simulink model "c00004M_harness"  (R2018a)
settings: Solver=ode3  StartTime=0.0  StopTime=10.0  RelTol=1e-3  EnableMultiTasking=on
undefined symbols (not defined in the file): b, DiscIntNeverNeededParam, J, K, L, PosMinimaW3, PosMinimaW4, R, sigbuilder_block
(part 22 of 74)

== system c00004M_harness/M132/Cyber ==
  note: Sensors
  note: Inputs For Window1
  note: Inputs for Window 2
  note: Inputs for window 3
  note: Inputs for window 4
  note: Users
  note: Users
  note: Sensors
  note: Users
  note: Sensors
  note: Users
  note: Sensors
  note: USERS
      | ---------------------------------
      | 0: None
      | 1: Ventana Arriba
      | 2: Ventana hasta arriba
      | 3: Ventana abajo
      | 4: Ventana hasta abajo
  note: 1: SUBE
      | 0: PARADO
      | -1 BAJA
  note: D = Driver (W1)
      | P1 = Passenger 1 (W2)
      | P2 = Passenger 2 (W3)
      | P3 = Passenger 3 (W4)
      | O = Obstacle
      | C = Control
      | Pri = Prioritizer
      | LD = LockDriver
      | PosW = PositionWindow
      | WL = WindowLogic
      | OW = ObstacleWindow
      | CWXC = ControlWindowXCentralized
      | S = Sensor
      | L = Lock
      | WPos = WindowPosition
      | M = Memory
      | InW = InputWindow
      | WIn = WindowInput
  PosW1 : Inport
  PosW2 : Inport  Port=2
  PosW3 : Inport  Port=3
  PosW4 : Inport  Port=4
  DW1 : Inport  Port=5
  DW3 : Inport  Port=6
  DW4 : Inport  Port=7
  P1W2 : Inport  Port=8
  P2W3 : Inport  Port=9
  P1W3 : Inport  Port=10
  P3W4 : Inport  Port=11
  P1W4 : Inport  Port=12
  OW1 : Inport  Port=13
  OW2 : Inport  Port=14
  OW3 : Inport  Port=15
  OW4 : Inport  Port=16
  CW1C : Inport  Port=17
  CW3C : Inport  Port=18
  CW4C : Inport  Port=19
  Pri1 : Subsystem
  Pri3 : Subsystem
  Pri4 : Subsystem
  WL : Subsystem
  WL1 : Subsystem
  WL2 : Subsystem
  WL3 : Subsystem
  W1 : Outport
  W2 : Outport  Port=2
  W3 : Outport  Port=3
  W4 : Outport  Port=4
  wires:
  CW4C/1 -> Pri4/4(CW4C)
  CW3C/1 -> Pri1/4(CW3C)
  CW1C/1 -> Pri3/2(CW1C)
  Pri3/1(User) -> WL/2(User)
  WL3/1(WindowLogicOutput) -> W4/1
  WL2/1(WindowLogicOutput) -> W3/1
  Pri4/1(User) -> WL3/2(User)
  OW4/1 -> WL3/3(OW)
  PosW4/1 -> WL3/1(WPos)
  P1W4/1 -> Pri4/3(P1)
  P3W4/1 -> Pri4/2(P)
  DW4/1 -> Pri4/1(D)
  P1W3/1 -> Pri1/3(P1)
  P2W3/1 -> Pri1/2(P)
  DW3/1 -> Pri1/1(D)
  OW3/1 -> WL2/3(OW)
  PosW3/1 -> WL2/1(WPos)
  Pri1/1(User) -> WL2/2(User)
  WL1/1(WindowLogicOutput) -> W2/1
  OW2/1 -> WL1/3(OW)
  PosW2/1 -> WL1/1(WPos)
  WL/1(WindowLogicOutput) -> W1/1
  DW1/1 -> Pri3/1(D)
  OW1/1 -> WL/3(OW)
  PosW1/1 -> WL/1(WPos)
  P1W2/1 -> WL1/2(User)

== system c00004M_harness/M132/Physical ==
  InW1 : Inport
  InW2 : Inport  Port=2
  InW3 : Inport  Port=3
  InW4 : Inport  Port=4
  W : Subsystem
  W5 : Subsystem
  W6 : Subsystem
  W7 : Subsystem
  W1 : Outport
  W2 : Outport  Port=2
  W3 : Outport  Port=3
  W4 : Outport  Port=4
  wires:
  W7/1(WPos) -> W4/1
  W6/1(WPos) -> W3/1
  W5/1(WPos) -> W2/1
  W/1(WPos) -> W1/1
  InW4/1 -> W7/1(WIn)
  InW3/1 -> W6/1(WIn)
  InW2/1 -> W5/1(WIn)
  InW1/1 -> W/1(WIn)

== system c00004M_harness/M132/S1 ==
  PhyMeasure : Inport
  SensorOut : Outport
  wires:
  PhyMeasure/1 -> SensorOut/1

== system c00004M_harness/M132/S2 ==
  PhyMeasure : Inport
  SensorOut : Outport
  wires:
  PhyMeasure/1 -> SensorOut/1

== system c00004M_harness/M132/S3 ==
  PhyMeasure : Inport
  SensorOut : Outport
  wires:
  PhyMeasure/1 -> SensorOut/1

== system c00004M_harness/M132/S4 ==
  PhyMeasure : Inport
  SensorOut : Outport
  wires:
  PhyMeasure/1 -> SensorOut/1

== system c00004M_harness/M133/Cyber ==
  note: Sensors
  note: Inputs For Window1
  note: Inputs for Window 2
  note: Inputs for window 3
  note: Inputs for window 4
  note: Users
  note: Users
  note: Sensors
  note: Users
  note: Sensors
  note: Users
  note: Sensors
  note: USERS
      | ---------------------------------
      | 0: None
      | 1: Ventana Arriba
      | 2: Ventana hasta arriba
      | 3: Ventana abajo
      | 4: Ventana hasta abajo
  note: 1: SUBE
      | 0: PARADO
      | -1 BAJA
  note: D = Driver (W1)
      | P1 = Passenger 1 (W2)
      | P2 = Passenger 2 (W3)
      | P3 = Passenger 3 (W4)
      | O = Obstacle
      | C = Control
      | Pri = Prioritizer
      | LD = LockDriver
      | PosW = PositionWindow
      | WL = WindowLogic
      | OW = ObstacleWindow
      | CWXC = ControlWindowXCentralized
      | S = Sensor
      | L = Lock
      | WPos = WindowPosition
      | M = Memory
      | InW = InputWindow
      | WIn = WindowInput
  PosW1 : Inport
  PosW2 : Inport  Port=2
  PosW3 : Inport  Port=3
  PosW4 : Inport  Port=4
  DW1 : Inport  Port=5
  DW3 : Inport  Port=6
  DW4 : Inport  Port=7
  P1W2 : Inport  Port=8
  P2W3 : Inport  Port=9
  P1W3 : Inport  Port=10
  P3W4 : Inport  Port=11
  P1W4 : Inport  Port=12
  OW1 : Inport  Port=13
  OW2 : Inport  Port=14
  OW3 : Inport  Port=15
  OW4 : Inport  Port=16
  CW1C : Inport  Port=17
  CW3C : Inport  Port=18
  CW4C : Inport  Port=19
  Pri1 : Subsystem
  Pri3 : Subsystem
  Pri4 : Subsystem
  WL : Subsystem
  WL1 : Subsystem
  WL2 : Subsystem
  WL3 : Subsystem
  W1 : Outport
  W2 : Outport  Port=2
  W3 : Outport  Port=3
  W4 : Outport  Port=4
  wires:
  CW4C/1 -> Pri4/4(CW4C)
  CW3C/1 -> Pri1/4(CW3C)
  CW1C/1 -> Pri3/2(CW1C)
  Pri3/1(User) -> WL/2(User)
  WL3/1(WindowLogicOutput) -> W4/1
  WL2/1(WindowLogicOutput) -> W3/1
  Pri4/1(User) -> WL3/2(User)
  OW4/1 -> WL3/3(OW)
  PosW4/1 -> WL3/1(WPos)
  P1W4/1 -> Pri4/3(P1)
  P3W4/1 -> Pri4/2(P)
  DW4/1 -> Pri4/1(D)
  P1W3/1 -> Pri1/3(P1)
  P2W3/1 -> Pri1/2(P)
  DW3/1 -> Pri1/1(D)
  OW3/1 -> WL2/3(OW)
  PosW3/1 -> WL2/1(WPos)
  Pri1/1(User) -> WL2/2(User)
  WL1/1(WindowLogicOutput) -> W2/1
  OW2/1 -> WL1/3(OW)
  PosW2/1 -> WL1/1(WPos)
  WL/1(WindowLogicOutput) -> W1/1
  DW1/1 -> Pri3/1(D)
  OW1/1 -> WL/3(OW)
  PosW1/1 -> WL/1(WPos)
  P1W2/1 -> WL1/2(User)

== system c00004M_harness/M133/Physical ==
  InW1 : Inport
  InW2 : Inport  Port=2
  InW3 : Inport  Port=3
  InW4 : Inport  Port=4
  W : Subsystem
  W5 : Subsystem
  W6 : Subsystem
  W7 : Subsystem
  W1 : Outport
  W2 : Outport  Port=2
  W3 : Outport  Port=3
  W4 : Outport  Port=4
  wires:
  W7/1(WPos) -> W4/1
  W6/1(WPos) -> W3/1
  W5/1(WPos) -> W2/1
  W/1(WPos) -> W1/1
  InW4/1 -> W7/1(WIn)
  InW3/1 -> W6/1(WIn)
  InW2/1 -> W5/1(WIn)
  InW1/1 -> W/1(WIn)

== system c00004M_harness/M133/S1 ==
  PhyMeasure : Inport
  SensorOut : Outport
  wires:
  PhyMeasure/1 -> SensorOut/1

== system c00004M_harness/M133/S2 ==
  PhyMeasure : Inport
  SensorOut : Outport
  wires:
  PhyMeasure/1 -> SensorOut/1

== system c00004M_harness/M133/S3 ==
  PhyMeasure : Inport
  SensorOut : Outport
  wires:
  PhyMeasure/1 -> SensorOut/1

== system c00004M_harness/M133/S4 ==
  PhyMeasure : Inport
  SensorOut : Outport
  wires:
  PhyMeasure/1 -> SensorOut/1

== system c00004M_harness/M134/Cyber ==
  note: Sensors
  note: Inputs For Window1
  note: Inputs for Window 2
  note: Inputs for window 3
  note: Inputs for window 4
  note: Users
  note: Users
  note: Sensors
  note: Users
  note: Sensors
  note: Users
  note: Sensors
  note: USERS
      | ---------------------------------
      | 0: None
      | 1: Ventana Arriba
      | 2: Ventana hasta arriba
      | 3: Ventana abajo
      | 4: Ventana hasta abajo
  note: 1: SUBE
      | 0: PARADO
      | -1 BAJA
  note: D = Driver (W1)
      | P1 = Passenger 1 (W2)
      | P2 = Passenger 2 (W3)
      | P3 = Passenger 3 (W4)
      | O = Obstacle
      | C = Control
      | Pri = Prioritizer
      | LD = LockDriver
      | PosW = PositionWindow
      | WL = WindowLogic
      | OW = ObstacleWindow
      | CWXC = ControlWindowXCentralized
      | S = Sensor
      | L = Lock
      | WPos = WindowPosition
      | M = Memory
      | InW = InputWindow
      | WIn = WindowInput
  PosW1 : Inport
  PosW2 : Inport  Port=2
  PosW3 : Inport  Port=3
  PosW4 : Inport  Port=4
  DW1 : Inport  Port=5
  DW3 : Inport  Port=6
  DW4 : Inport  Port=7
  P1W2 : Inport  Port=8
  P2W3 : Inport  Port=9
  P1W3 : Inport  Port=10
  P3W4 : Inport  Port=11
  P1W4 : Inport  Port=12
  OW1 : Inport  Port=13
  OW2 : Inport  Port=14
  OW3 : Inport  Port=15
  OW4 : Inport  Port=16
  CW1C : Inport  Port=17
  CW3C : Inport  Port=18
  CW4C : Inport  Port=19
  Pri1 : Subsystem
  Pri3 : Subsystem
  Pri4 : Subsystem
  WL : Subsystem
  WL1 : Subsystem
  WL2 : Subsystem
  WL3 : Subsystem
  W1 : Outport
  W2 : Outport  Port=2
  W3 : Outport  Port=3
  W4 : Outport  Port=4
  wires:
  CW4C/1 -> Pri4/4(CW4C)
  CW3C/1 -> Pri1/4(CW3C)
  CW1C/1 -> Pri3/2(CW1C)
  Pri3/1(User) -> WL/2(User)
  WL3/1(WindowLogicOutput) -> W4/1
  WL2/1(WindowLogicOutput) -> W3/1
  Pri4/1(User) -> WL3/2(User)
  OW4/1 -> WL3/3(OW)
  PosW4/1 -> WL3/1(WPos)
  P1W4/1 -> Pri4/3(P1)
  P3W4/1 -> Pri4/2(P)
  DW4/1 -> Pri4/1(D)
  P1W3/1 -> Pri1/3(P1)
  P2W3/1 -> Pri1/2(P)
  DW3/1 -> Pri1/1(D)
  OW3/1 -> WL2/3(OW)
  PosW3/1 -> WL2/1(WPos)
  Pri1/1(User) -> WL2/2(User)
  WL1/1(WindowLogicOutput) -> W2/1
  OW2/1 -> WL1/3(OW)
  PosW2/1 -> WL1/1(WPos)
  WL/1(WindowLogicOutput) -> W1/1
  DW1/1 -> Pri3/1(D)
  OW1/1 -> WL/3(OW)
  PosW1/1 -> WL/1(WPos)
  P1W2/1 -> WL1/2(User)

== system c00004M_harness/M134/Physical ==
  InW1 : Inport
  InW2 : Inport  Port=2
  InW3 : Inport  Port=3
  InW4 : Inport  Port=4
  W : Subsystem
  W5 : Subsystem
  W6 : Subsystem
  W7 : Subsystem
  W1 : Outport
  W2 : Outport  Port=2
  W3 : Outport  Port=3
  W4 : Outport  Port=4
  wires:
  W7/1(WPos) -> W4/1
  W6/1(WPos) -> W3/1
  W5/1(WPos) -> W2/1
  W/1(WPos) -> W1/1
  InW4/1 -> W7/1(WIn)
  InW3/1 -> W6/1(WIn)
  InW2/1 -> W5/1(WIn)
  InW1/1 -> W/1(WIn)

== system c00004M_harness/M134/S1 ==
  PhyMeasure : Inport
  SensorOut : Outport
  wires:
  PhyMeasure/1 -> SensorOut/1

== system c00004M_harness/M134/S2 ==
  PhyMeasure : Inport
  SensorOut : Outport
  wires:
  PhyMeasure/1 -> SensorOut/1

== system c00004M_harness/M134/S3 ==
  PhyMeasure : Inport
  SensorOut : Outport
  wires:
  PhyMeasure/1 -> SensorOut/1

== system c00004M_harness/M134/S4 ==
  PhyMeasure : Inport
  SensorOut : Outport
  wires:
  PhyMeasure/1 -> SensorOut/1

== system c00004M_harness/M135/Cyber ==
  note: Sensors
  note: Inputs For Window1
  note: Inputs for Window 2
  note: Inputs for window 3
  note: Inputs for window 4
  note: Users
  note: Users
  note: Sensors
  note: Users
  note: Sensors
  note: Users
  note: Sensors
  note: USERS
      | ---------------------------------
      | 0: None
      | 1: Ventana Arriba
      | 2: Ventana hasta arriba
      | 3: Ventana abajo
      | 4: Ventana hasta abajo
  note: 1: SUBE
      | 0: PARADO
      | -1 BAJA
  note: D = Driver (W1)
      | P1 = Passenger 1 (W2)
      | P2 = Passenger 2 (W3)
      | P3 = Passenger 3 (W4)
      | O = Obstacle
      | C = Control
      | Pri = Prioritizer
      | LD = LockDriver
      | PosW = PositionWindow
      | WL = WindowLogic
      | OW = ObstacleWindow
      | CWXC = ControlWindowXCentralized
      | S = Sensor
      | L = Lock
      | WPos = WindowPosition
      | M = Memory
      | InW = InputWindow
      | WIn = WindowInput
  PosW1 : Inport
  PosW2 : Inport  Port=2
  PosW3 : Inport  Port=3
  PosW4 : Inport  Port=4
  DW1 : Inport  Port=5
  DW3 : Inport  Port=6
  DW4 : Inport  Port=7
  P1W2 : Inport  Port=8
  P2W3 : Inport  Port=9
  P1W3 : Inport  Port=10
  P3W4 : Inport  Port=11
  P1W4 : Inport  Port=12
  OW1 : Inport  Port=13
  OW2 : Inport  Port=14
  OW3 : Inport  Port=15
  OW4 : Inport  Port=16
  CW1C : Inport  Port=17
  CW3C : Inport  Port=18
  CW4C : Inport  Port=19
  Pri1 : Subsystem
  Pri3 : Subsystem
  Pri4 : Subsystem
  WL : Subsystem
  WL1 : Subsystem
  WL2 : Subsystem
  WL3 : Subsystem
  W1 : Outport
  W2 : Outport  Port=2
  W3 : Outport  Port=3
  W4 : Outport  Port=4
  wires:
  CW4C/1 -> Pri4/4(CW4C)
  CW3C/1 -> Pri1/4(CW3C)
  CW1C/1 -> Pri3/2(CW1C)
  Pri3/1(User) -> WL/2(User)
  WL3/1(WindowLogicOutput) -> W4/1
  WL2/1(WindowLogicOutput) -> W3/1
  Pri4/1(User) -> WL3/2(User)
  OW4/1 -> WL3/3(OW)
  PosW4/1 -> WL3/1(WPos)
  P1W4/1 -> Pri4/3(P1)
  P3W4/1 -> Pri4/2(P)
  DW4/1 -> Pri4/1(D)
  P1W3/1 -> Pri1/3(P1)
  P2W3/1 -> Pri1/2(P)
  DW3/1 -> Pri1/1(D)
  OW3/1 -> WL2/3(OW)
  PosW3/1 -> WL2/1(WPos)
  Pri1/1(User) -> WL2/2(User)
  WL1/1(WindowLogicOutput) -> W2/1
  OW2/1 -> WL1/3(OW)
  PosW2/1 -> WL1/1(WPos)
  WL/1(WindowLogicOutput) -> W1/1
  DW1/1 -> Pri3/1(D)
  OW1/1 -> WL/3(OW)
  PosW1/1 -> WL/1(WPos)
  P1W2/1 -> WL1/2(User)

== system c00004M_harness/M135/Physical ==
  InW1 : Inport
  InW2 : Inport  Port=2
  InW3 : Inport  Port=3
  InW4 : Inport  Port=4
  W : Subsystem
  W5 : Subsystem
  W6 : Subsystem
  W7 : Subsystem
  W1 : Outport
  W2 : Outport  Port=2
  W3 : Outport  Port=3
  W4 : Outport  Port=4
  wires:
  W7/1(WPos) -> W4/1
  W6/1(WPos) -> W3/1
  W5/1(WPos) -> W2/1
  W/1(WPos) -> W1/1
  InW4/1 -> W7/1(WIn)
  InW3/1 -> W6/1(WIn)
  InW2/1 -> W5/1(WIn)
  InW1/1 -> W/1(WIn)

== system c00004M_harness/M135/S1 ==
  PhyMeasure : Inport
  SensorOut : Outport
  wires:
  PhyMeasure/1 -> SensorOut/1

== system c00004M_harness/M135/S2 ==
  PhyMeasure : Inport
  SensorOut : Outport
  wires:
  PhyMeasure/1 -> SensorOut/1

== system c00004M_harness/M135/S3 ==
  PhyMeasure : Inport
  SensorOut : Outport
  wires:
  PhyMeasure/1 -> SensorOut/1

== system c00004M_harness/M135/S4 ==
  PhyMeasure : Inport
  SensorOut : Outport
  wires:
  PhyMeasure/1 -> SensorOut/1

== system c00004M_harness/M136/Cyber ==
  note: Sensors
  note: Inputs For Window1
  note: Inputs for Window 2
  note: Inputs for window 3
  note: Inputs for window 4
  note: Users
  note: Users
  note: Sensors
  note: Users
  note: Sensors
  note: Users
  note: Sensors
  note: USERS
      | ---------------------------------
      | 0: None
      | 1: Ventana Arriba
      | 2: Ventana hasta arriba
      | 3: Ventana abajo
      | 4: Ventana hasta abajo
  note: 1: SUBE
      | 0: PARADO
      | -1 BAJA
  note: D = Driver (W1)
      | P1 = Passenger 1 (W2)
      | P2 = Passenger 2 (W3)
      | P3 = Passenger 3 (W4)
      | O = Obstacle
      | C = Control
      | Pri = Prioritizer
      | LD = LockDriver
      | PosW = PositionWindow
      | WL = WindowLogic
      | OW = ObstacleWindow
      | CWXC = ControlWindowXCentralized
      | S = Sensor
      | L = Lock
      | WPos = WindowPosition
      | M = Memory
      | InW = InputWindow
      | WIn = WindowInput
  PosW1 : Inport
  PosW2 : Inport  Port=2
  PosW3 : Inport  Port=3
  PosW4 : Inport  Port=4
  DW1 : Inport  Port=5
  DW3 : Inport  Port=6
  DW4 : Inport  Port=7
  P1W2 : Inport  Port=8
  P2W3 : Inport  Port=9
  P1W3 : Inport  Port=10
  P3W4 : Inport  Port=11
  P1W4 : Inport  Port=12
  OW1 : Inport  Port=13
  OW2 : Inport  Port=14
  OW3 : Inport  Port=15
  OW4 : Inport  Port=16
  CW1C : Inport  Port=17
  CW3C : Inport  Port=18
  CW4C : Inport  Port=19
  Pri1 : Subsystem
  Pri3 : Subsystem
  Pri4 : Subsystem
  WL : Subsystem
  WL1 : Subsystem
  WL2 : Subsystem
  WL3 : Subsystem
  W1 : Outport
  W2 : Outport  Port=2
  W3 : Outport  Port=3
  W4 : Outport  Port=4
  wires:
  CW4C/1 -> Pri4/4(CW4C)
  CW3C/1 -> Pri1/4(CW3C)
  CW1C/1 -> Pri3/2(CW1C)
  Pri3/1(User) -> WL/2(User)
  WL3/1(WindowLogicOutput) -> W4/1
  WL2/1(WindowLogicOutput) -> W3/1
  Pri4/1(User) -> WL3/2(User)
  OW4/1 -> WL3/3(OW)
  PosW4/1 -> WL3/1(WPos)
  P1W4/1 -> Pri4/3(P1)
  P3W4/1 -> Pri4/2(P)
  DW4/1 -> Pri4/1(D)
  P1W3/1 -> Pri1/3(P1)
  P2W3/1 -> Pri1/2(P)
  DW3/1 -> Pri1/1(D)
  OW3/1 -> WL2/3(OW)
  PosW3/1 -> WL2/1(WPos)
  Pri1/1(User) -> WL2/2(User)
  WL1/1(WindowLogicOutput) -> W2/1
  OW2/1 -> WL1/3(OW)
  PosW2/1 -> WL1/1(WPos)
  WL/1(WindowLogicOutput) -> W1/1
  DW1/1 -> Pri3/1(D)
  OW1/1 -> WL/3(OW)
  PosW1/1 -> WL/1(WPos)
  P1W2/1 -> WL1/2(User)

== system c00004M_harness/M136/Physical ==
  InW1 : Inport
  InW2 : Inport  Port=2
  InW3 : Inport  Port=3
  InW4 : Inport  Port=4
  W : Subsystem
  W5 : Subsystem
  W6 : Subsystem
  W7 : Subsystem
  W1 : Outport
  W2 : Outport  Port=2
  W3 : Outport  Port=3
  W4 : Outport  Port=4
  wires:
  W7/1(WPos) -> W4/1
  W6/1(WPos) -> W3/1
  W5/1(WPos) -> W2/1
  W/1(WPos) -> W1/1
  InW4/1 -> W7/1(WIn)
  InW3/1 -> W6/1(WIn)
  InW2/1 -> W5/1(WIn)
  InW1/1 -> W/1(WIn)

== system c00004M_harness/M136/S1 ==
  PhyMeasure : Inport
  SensorOut : Outport
  wires:
  PhyMeasure/1 -> SensorOut/1

== system c00004M_harness/M136/S2 ==
  PhyMeasure : Inport
  SensorOut : Outport
  wires:
  PhyMeasure/1 -> SensorOut/1

== system c00004M_harness/M136/S3 ==
  PhyMeasure : Inport
  SensorOut : Outport
  wires:
  PhyMeasure/1 -> SensorOut/1

== system c00004M_harness/M136/S4 ==
  PhyMeasure : Inport
  SensorOut : Outport
  wires:
  PhyMeasure/1 -> SensorOut/1

== system c00004M_harness/M137/Cyber ==
  note: Sensors
  note: Inputs For Window1
  note: Inputs for Window 2
  note: Inputs for window 3
  note: Inputs for window 4
  note: Users
  note: Users
  note: Sensors
  note: Users
  note: Sensors
  note: Users
  note: Sensors
  note: USERS
      | ---------------------------------
      | 0: None
      | 1: Ventana Arriba
      | 2: Ventana hasta arriba
      | 3: Ventana abajo
      | 4: Ventana hasta abajo
  note: 1: SUBE
      | 0: PARADO
      | -1 BAJA
  note: D = Driver (W1)
      | P1 = Passenger 1 (W2)
      | P2 = Passenger 2 (W3)
      | P3 = Passenger 3 (W4)
      | O = Obstacle
      | C = Control
      | Pri = Prioritizer
      | LD = LockDriver
      | PosW = PositionWindow
      | WL = WindowLogic
      | OW = ObstacleWindow
      | CWXC = ControlWindowXCentralized
      | S = Sensor
      | L = Lock
      | WPos = WindowPosition
      | M = Memory
      | InW = InputWindow
      | WIn = WindowInput
  PosW1 : Inport
  PosW2 : Inport  Port=2
  PosW3 : Inport  Port=3
  PosW4 : Inport  Port=4
  DW1 : Inport  Port=5
  DW3 : Inport  Port=6
  DW4 : Inport  Port=7
  P1W2 : Inport  Port=8
  P2W3 : Inport  Port=9
  P1W3 : Inport  Port=10
  P3W4 : Inport  Port=11
  P1W4 : Inport  Port=12
  OW1 : Inport  Port=13
  OW2 : Inport  Port=14
  OW3 : Inport  Port=15
  OW4 : Inport  Port=16
  CW1C : Inport  Port=17
  CW3C : Inport  Port=18
  CW4C : Inport  Port=19
  Pri1 : Subsystem
  Pri3 : Subsystem
  Pri4 : Subsystem
  WL : Subsystem
  WL1 : Subsystem
  WL2 : Subsystem
  WL3 : Subsystem
  W1 : Outport
  W2 : Outport  Port=2
  W3 : Outport  Port=3
  W4 : Outport  Port=4
  wires:
  CW4C/1 -> Pri4/4(CW4C)
  CW3C/1 -> Pri1/4(CW3C)
  CW1C/1 -> Pri3/2(CW1C)
  Pri3/1(User) -> WL/2(User)
  WL3/1(WindowLogicOutput) -> W4/1
  WL2/1(WindowLogicOutput) -> W3/1
  Pri4/1(User) -> WL3/2(User)
  OW4/1 -> WL3/3(OW)
  PosW4/1 -> WL3/1(WPos)
  P1W4/1 -> Pri4/3(P1)
  P3W4/1 -> Pri4/2(P)
  DW4/1 -> Pri4/1(D)
  P1W3/1 -> Pri1/3(P1)
  P2W3/1 -> Pri1/2(P)
  DW3/1 -> Pri1/1(D)
  OW3/1 -> WL2/3(OW)
  PosW3/1 -> WL2/1(WPos)
  Pri1/1(User) -> WL2/2(User)
  WL1/1(WindowLogicOutput) -> W2/1
  OW2/1 -> WL1/3(OW)
  PosW2/1 -> WL1/1(WPos)
  WL/1(WindowLogicOutput) -> W1/1
  DW1/1 -> Pri3/1(D)
  OW1/1 -> WL/3(OW)
  PosW1/1 -> WL/1(WPos)
  P1W2/1 -> WL1/2(User)

== system c00004M_harness/M137/Physical ==
  InW1 : Inport
  InW2 : Inport  Port=2
  InW3 : Inport  Port=3
  InW4 : Inport  Port=4
  W : Subsystem
  W5 : Subsystem
  W6 : Subsystem
  W7 : Subsystem
  W1 : Outport
  W2 : Outport  Port=2
  W3 : Outport  Port=3
  W4 : Outport  Port=4
  wires:
  W7/1(WPos) -> W4/1
  W6/1(WPos) -> W3/1
  W5/1(WPos) -> W2/1
  W/1(WPos) -> W1/1
  InW4/1 -> W7/1(WIn)
  InW3/1 -> W6/1(WIn)
  InW2/1 -> W5/1(WIn)
  InW1/1 -> W/1(WIn)

== system c00004M_harness/M137/S1 ==
  PhyMeasure : Inport
  SensorOut : Outport
  wires:
  PhyMeasure/1 -> SensorOut/1

== system c00004M_harness/M137/S2 ==
  PhyMeasure : Inport
  SensorOut : Outport
  wires:
  PhyMeasure/1 -> SensorOut/1

== system c00004M_harness/M137/S3 ==
  PhyMeasure : Inport
  SensorOut : Outport
  wires:
  PhyMeasure/1 -> SensorOut/1

== system c00004M_harness/M137/S4 ==
  PhyMeasure : Inport
  SensorOut : Outport
  wires:
  PhyMeasure/1 -> SensorOut/1

== system c00004M_harness/M138/Cyber ==
  note: Sensors
  note: Inputs For Window1
  note: Inputs for Window 2
  note: Inputs for window 3
  note: Inputs for window 4
  note: Users
  note: Users
  note: Sensors
  note: Users
  note: Sensors
  note: Users
  note: Sensors
  note: USERS
      | ---------------------------------
      | 0: None
      | 1: Ventana Arriba
      | 2: Ventana hasta arriba
      | 3: Ventana abajo
      | 4: Ventana hasta abajo
  note: 1: SUBE
      | 0: PARADO
      | -1 BAJA
  note: D = Driver (W1)
      | P1 = Passenger 1 (W2)
      | P2 = Passenger 2 (W3)
      | P3 = Passenger 3 (W4)
      | O = Obstacle
      | C = Control
      | Pri = Prioritizer
      | LD = LockDriver
      | PosW = PositionWindow
      | WL = WindowLogic
      | OW = ObstacleWindow
      | CWXC = ControlWindowXCentralized
      | S = Sensor
      | L = Lock
      | WPos = WindowPosition
      | M = Memory
      | InW = InputWindow
      | WIn = WindowInput
  PosW1 : Inport
  PosW2 : Inport  Port=2
  PosW3 : Inport  Port=3
  PosW4 : Inport  Port=4
  DW1 : Inport  Port=5
  DW3 : Inport  Port=6
  DW4 : Inport  Port=7
  P1W2 : Inport  Port=8
  P2W3 : Inport  Port=9
  P1W3 : Inport  Port=10
  P3W4 : Inport  Port=11
  P1W4 : Inport  Port=12
  OW1 : Inport  Port=13
  OW2 : Inport  Port=14
  OW3 : Inport  Port=15
  OW4 : Inport  Port=16
  CW1C : Inport  Port=17
  CW3C : Inport  Port=18
  CW4C : Inport  Port=19
  Pri1 : Subsystem
  Pri3 : Subsystem
  Pri4 : Subsystem
  WL : Subsystem
  WL1 : Subsystem
  WL2 : Subsystem
  WL3 : Subsystem
  W1 : Outport
  W2 : Outport  Port=2
  W3 : Outport  Port=3
  W4 : Outport  Port=4
  wires:
  CW4C/1 -> Pri4/4(CW4C)
  CW3C/1 -> Pri1/4(CW3C)
  CW1C/1 -> Pri3/2(CW1C)
  Pri3/1(User) -> WL/2(User)
  WL3/1(WindowLogicOutput) -> W4/1
  WL2/1(WindowLogicOutput) -> W3/1
  Pri4/1(User) -> WL3/2(User)
  OW4/1 -> WL3/3(OW)
  PosW4/1 -> WL3/1(WPos)
  P1W4/1 -> Pri4/3(P1)
  P3W4/1 -> Pri4/2(P)
  DW4/1 -> Pri4/1(D)
  P1W3/1 -> Pri1/3(P1)
  P2W3/1 -> Pri1/2(P)
  DW3/1 -> Pri1/1(D)
  OW3/1 -> WL2/3(OW)
  PosW3/1 -> WL2/1(WPos)
  Pri1/1(User) -> WL2/2(User)
  WL1/1(WindowLogicOutput) -> W2/1
  OW2/1 -> WL1/3(OW)
  PosW2/1 -> WL1/1(WPos)
  WL/1(WindowLogicOutput) -> W1/1
  DW1/1 -> Pri3/1(D)
  OW1/1 -> WL/3(OW)
  PosW1/1 -> WL/1(WPos)
  P1W2/1 -> WL1/2(User)

== system c00004M_harness/M138/Physical ==
  InW1 : Inport
  InW2 : Inport  Port=2
  InW3 : Inport  Port=3
  InW4 : Inport  Port=4
  W : Subsystem
  W5 : Subsystem
  W6 : Subsystem
  W7 : Subsystem
  W1 : Outport
  W2 : Outport  Port=2
  W3 : Outport  Port=3
  W4 : Outport  Port=4
  wires:
  W7/1(WPos) -> W4/1
  W6/1(WPos) -> W3/1
  W5/1(WPos) -> W2/1
  W/1(WPos) -> W1/1
  InW4/1 -> W7/1(WIn)
  InW3/1 -> W6/1(WIn)
  InW2/1 -> W5/1(WIn)
  InW1/1 -> W/1(WIn)

== system c00004M_harness/M138/S1 ==
  PhyMeasure : Inport
  SensorOut : Outport
  wires:
  PhyMeasure/1 -> SensorOut/1

== system c00004M_harness/M138/S2 ==
  PhyMeasure : Inport
  SensorOut : Outport
  wires:
  PhyMeasure/1 -> SensorOut/1

== system c00004M_harness/M138/S3 ==
  PhyMeasure : Inport
  SensorOut : Outport
  wires:
  PhyMeasure/1 -> SensorOut/1

== system c00004M_harness/M138/S4 ==
  PhyMeasure : Inport
  SensorOut : Outport
  wires:
  PhyMeasure/1 -> SensorOut/1

== system c00004M_harness/M139/Cyber ==
  note: Sensors
  note: Inputs For Window1
  note: Inputs for Window 2
  note: Inputs for window 3
  note: Inputs for window 4
  note: Users
  note: Users
  note: Sensors
  note: Users
  note: Sensors
  note: Users
  note: Sensors
  note: USERS
      | ---------------------------------
      | 0: None
      | 1: Ventana Arriba
      | 2: Ventana hasta arriba
      | 3: Ventana abajo
      | 4: Ventana hasta abajo
  note: 1: SUBE
      | 0: PARADO
      | -1 BAJA
  note: D = Driver (W1)
      | P1 = Passenger 1 (W2)
      | P2 = Passenger 2 (W3)
      | P3 = Passenger 3 (W4)
      | O = Obstacle
      | C = Control
      | Pri = Prioritizer
      | LD = LockDriver
      | PosW = PositionWindow
      | WL = WindowLogic
      | OW = ObstacleWindow
      | CWXC = ControlWindowXCentralized
      | S = Sensor
      | L = Lock
      | WPos = WindowPosition
      | M = Memory
      | InW = InputWindow
      | WIn = WindowInput
  PosW1 : Inport
  PosW2 : Inport  Port=2
  PosW3 : Inport  Port=3
  PosW4 : Inport  Port=4
  DW1 : Inport  Port=5
  DW3 : Inport  Port=6
  DW4 : Inport  Port=7
  P1W2 : Inport  Port=8
  P2W3 : Inport  Port=9
  P1W3 : Inport  Port=10
  P3W4 : Inport  Port=11
  P1W4 : Inport  Port=12
  OW1 : Inport  Port=13
  OW2 : Inport  Port=14
  OW3 : Inport  Port=15
  OW4 : Inport  Port=16
  CW1C : Inport  Port=17
  CW3C : Inport  Port=18
  CW4C : Inport  Port=19
  Pri1 : Subsystem
  Pri3 : Subsystem
  Pri4 : Subsystem
  WL : Subsystem
  WL1 : Subsystem
  WL2 : Subsystem
  WL3 : Subsystem
  W1 : Outport
  W2 : Outport  Port=2
  W3 : Outport  Port=3
  W4 : Outport  Port=4
  wires:
  CW4C/1 -> Pri4/4(CW4C)
  CW3C/1 -> Pri1/4(CW3C)
  CW1C/1 -> Pri3/2(CW1C)
  Pri3/1(User) -> WL/2(User)
  WL3/1(WindowLogicOutput) -> W4/1
  WL2/1(WindowLogicOutput) -> W3/1
  Pri4/1(User) -> WL3/2(User)
  OW4/1 -> WL3/3(OW)
  PosW4/1 -> WL3/1(WPos)
  P1W4/1 -> Pri4/3(P1)
  P3W4/1 -> Pri4/2(P)
  DW4/1 -> Pri4/1(D)
  P1W3/1 -> Pri1/3(P1)
  P2W3/1 -> Pri1/2(P)
  DW3/1 -> Pri1/1(D)
  OW3/1 -> WL2/3(OW)
  PosW3/1 -> WL2/1(WPos)
  Pri1/1(User) -> WL2/2(User)
  WL1/1(WindowLogicOutput) -> W2/1
  OW2/1 -> WL1/3(OW)
  PosW2/1 -> WL1/1(WPos)
  WL/1(WindowLogicOutput) -> W1/1
  DW1/1 -> Pri3/1(D)
  OW1/1 -> WL/3(OW)
  PosW1/1 -> WL/1(WPos)
  P1W2/1 -> WL1/2(User)

== system c00004M_harness/M139/Physical ==
  InW1 : Inport
  InW2 : Inport  Port=2
  InW3 : Inport  Port=3
  InW4 : Inport  Port=4
  W : Subsystem
  W5 : Subsystem
  W6 : Subsystem
  W7 : Subsystem
  W1 : Outport
  W2 : Outport  Port=2
  W3 : Outport  Port=3
  W4 : Outport  Port=4
  wires:
  W7/1(WPos) -> W4/1
  W6/1(WPos) -> W3/1
  W5/1(WPos) -> W2/1
  W/1(WPos) -> W1/1
  InW4/1 -> W7/1(WIn)
  InW3/1 -> W6/1(WIn)
  InW2/1 -> W5/1(WIn)
  InW1/1 -> W/1(WIn)

== system c00004M_harness/M139/S1 ==
  PhyMeasure : Inport
  SensorOut : Outport
  wires:
  PhyMeasure/1 -> SensorOut/1

== system c00004M_harness/M139/S2 ==
  PhyMeasure : Inport
  SensorOut : Outport
  wires:
  PhyMeasure/1 -> SensorOut/1

== system c00004M_harness/M139/S3 ==
  PhyMeasure : Inport
  SensorOut : Outport
  wires:
  PhyMeasure/1 -> SensorOut/1

== system c00004M_harness/M139/S4 ==
  PhyMeasure : Inport
  SensorOut : Outport
  wires:
  PhyMeasure/1 -> SensorOut/1

== system c00004M_harness/M140/Cyber ==
  note: Sensors
  note: Inputs For Window1
  note: Inputs for Window 2
  note: Inputs for window 3
  note: Inputs for window 4
  note: Users
  note: Users
  note: Sensors
  note: Users
  note: Sensors
  note: Users
  note: Sensors
  note: USERS
      | ---------------------------------
      | 0: None
      | 1: Ventana Arriba
      | 2: Ventana hasta arriba
      | 3: Ventana abajo
      | 4: Ventana hasta abajo
  note: 1: SUBE
      | 0: PARADO
      | -1 BAJA
  note: D = Driver (W1)
      | P1 = Passenger 1 (W2)
      | P2 = Passenger 2 (W3)
      | P3 = Passenger 3 (W4)
      | O = Obstacle
      | C = Control
      | Pri = Prioritizer
      | LD = LockDriver
      | PosW = PositionWindow
      | WL = WindowLogic
      | OW = ObstacleWindow
      | CWXC = ControlWindowXCentralized
      | S = Sensor
      | L = Lock
      | WPos = WindowPosition
      | M = Memory
      | InW = InputWindow
      | WIn = WindowInput
  PosW1 : Inport
  PosW2 : Inport  Port=2
  PosW3 : Inport  Port=3
  PosW4 : Inport  Port=4
  DW1 : Inport  Port=5
  DW3 : Inport  Port=6
  DW4 : Inport  Port=7
  P1W2 : Inport  Port=8
  P2W3 : Inport  Port=9
  P1W3 : Inport  Port=10
  P3W4 : Inport  Port=11
  P1W4 : Inport  Port=12
  OW1 : Inport  Port=13
  OW2 : Inport  Port=14
  OW3 : Inport  Port=15
  OW4 : Inport  Port=16
  CW1C : Inport  Port=17
  CW3C : Inport  Port=18
  CW4C : Inport  Port=19
  Pri1 : Subsystem
  Pri3 : Subsystem
  Pri4 : Subsystem
  WL : Subsystem
  WL1 : Subsystem
  WL2 : Subsystem
  WL3 : Subsystem
  W1 : Outport
  W2 : Outport  Port=2
  W3 : Outport  Port=3
  W4 : Outport  Port=4
  wires:
  CW4C/1 -> Pri4/4(CW4C)
  CW3C/1 -> Pri1/4(CW3C)
  CW1C/1 -> Pri3/2(CW1C)
  Pri3/1(User) -> WL/2(User)
  WL3/1(WindowLogicOutput) -> W4/1
  WL2/1(WindowLogicOutput) -> W3/1
  Pri4/1(User) -> WL3/2(User)
  OW4/1 -> WL3/3(OW)
  PosW4/1 -> WL3/1(WPos)
  P1W4/1 -> Pri4/3(P1)
  P3W4/1 -> Pri4/2(P)
  DW4/1 -> Pri4/1(D)
  P1W3/1 -> Pri1/3(P1)
  P2W3/1 -> Pri1/2(P)
  DW3/1 -> Pri1/1(D)
  OW3/1 -> WL2/3(OW)
  PosW3/1 -> WL2/1(WPos)
  Pri1/1(User) -> WL2/2(User)
  WL1/1(WindowLogicOutput) -> W2/1
  OW2/1 -> WL1/3(OW)
  PosW2/1 -> WL1/1(WPos)
  WL/1(WindowLogicOutput) -> W1/1
  DW1/1 -> Pri3/1(D)
  OW1/1 -> WL/3(OW)
  PosW1/1 -> WL/1(WPos)
  P1W2/1 -> WL1/2(User)

== system c00004M_harness/M140/Physical ==
  InW1 : Inport
  InW2 : Inport  Port=2
  InW3 : Inport  Port=3
  InW4 : Inport  Port=4
  W : Subsystem
  W5 : Subsystem
  W6 : Subsystem
  W7 : Subsystem
  W1 : Outport
  W2 : Outport  Port=2
  W3 : Outport  Port=3
  W4 : Outport  Port=4
  wires:
  W7/1(WPos) -> W4/1
  W6/1(WPos) -> W3/1
  W5/1(WPos) -> W2/1
  W/1(WPos) -> W1/1
  InW4/1 -> W7/1(WIn)
  InW3/1 -> W6/1(WIn)
  InW2/1 -> W5/1(WIn)
  InW1/1 -> W/1(WIn)

== system c00004M_harness/M140/S1 ==
  PhyMeasure : Inport
  SensorOut : Outport
  wires:
  PhyMeasure/1 -> SensorOut/1

== system c00004M_harness/M140/S2 ==
  PhyMeasure : Inport
  SensorOut : Outport
  wires:
  PhyMeasure/1 -> SensorOut/1

== system c00004M_harness/M140/S3 ==
  PhyMeasure : Inport
  SensorOut : Outport
  wires:
  PhyMeasure/1 -> SensorOut/1

== system c00004M_harness/M140/S4 ==
  PhyMeasure : Inport
  SensorOut : Outport
  wires:
  PhyMeasure/1 -> SensorOut/1

== system c00004M_harness/M141/Cyber ==
  note: Sensors
  note: Inputs For Window1
  note: Inputs for Window 2
  note: Inputs for window 3
  note: Inputs for window 4
  note: Users
  note: Users
  note: Sensors
  note: Users
  note: Sensors
  note: Users
  note: Sensors
  note: USERS
      | ---------------------------------
      | 0: None
      | 1: Ventana Arriba
      | 2: Ventana hasta arriba
      | 3: Ventana abajo
      | 4: Ventana hasta abajo
  note: 1: SUBE
      | 0: PARADO
      | -1 BAJA
  note: D = Driver (W1)
      | P1 = Passenger 1 (W2)
      | P2 = Passenger 2 (W3)
      | P3 = Passenger 3 (W4)
      | O = Obstacle
      | C = Control
      | Pri = Prioritizer
      | LD = LockDriver
      | PosW = PositionWindow
      | WL = WindowLogic
      | OW = ObstacleWindow
      | CWXC = ControlWindowXCentralized
      | S = Sensor
      | L = Lock
      | WPos = WindowPosition
      | M = Memory
      | InW = InputWindow
      | WIn = WindowInput
  PosW1 : Inport
  PosW2 : Inport  Port=2
  PosW3 : Inport  Port=3
  PosW4 : Inport  Port=4
  DW1 : Inport  Port=5
  DW3 : Inport  Port=6
  DW4 : Inport  Port=7
  P1W2 : Inport  Port=8
  P2W3 : Inport  Port=9
  P1W3 : Inport  Port=10
  P3W4 : Inport  Port=11
  P1W4 : Inport  Port=12
  OW1 : Inport  Port=13
  OW2 : Inport  Port=14
  OW3 : Inport  Port=15
  OW4 : Inport  Port=16
  CW1C : Inport  Port=17
  CW3C : Inport  Port=18
  CW4C : Inport  Port=19
  Pri1 : Subsystem
  Pri3 : Subsystem
  Pri4 : Subsystem
  WL : Subsystem
  WL1 : Subsystem
  WL2 : Subsystem
  WL3 : Subsystem
  W1 : Outport
  W2 : Outport  Port=2
  W3 : Outport  Port=3
  W4 : Outport  Port=4
  wires:
  CW4C/1 -> Pri4/4(CW4C)
  CW3C/1 -> Pri1/4(CW3C)
  CW1C/1 -> Pri3/2(CW1C)
  Pri3/1(User) -> WL/2(User)
  WL3/1(WindowLogicOutput) -> W4/1
  WL2/1(WindowLogicOutput) -> W3/1
  Pri4/1(User) -> WL3/2(User)
  OW4/1 -> WL3/3(OW)
  PosW4/1 -> WL3/1(WPos)
  P1W4/1 -> Pri4/3(P1)
  P3W4/1 -> Pri4/2(P)
  DW4/1 -> Pri4/1(D)
  P1W3/1 -> Pri1/3(P1)
  P2W3/1 -> Pri1/2(P)
  DW3/1 -> Pri1/1(D)
  OW3/1 -> WL2/3(OW)
  PosW3/1 -> WL2/1(WPos)
  Pri1/1(User) -> WL2/2(User)
  WL1/1(WindowLogicOutput) -> W2/1
  OW2/1 -> WL1/3(OW)
  PosW2/1 -> WL1/1(WPos)
  WL/1(WindowLogicOutput) -> W1/1
  DW1/1 -> Pri3/1(D)
  OW1/1 -> WL/3(OW)
  PosW1/1 -> WL/1(WPos)
  P1W2/1 -> WL1/2(User)

== system c00004M_harness/M141/Physical ==
  InW1 : Inport
  InW2 : Inport  Port=2
  InW3 : Inport  Port=3
  InW4 : Inport  Port=4
  W : Subsystem
  W5 : Subsystem
  W6 : Subsystem
  W7 : Subsystem
  W1 : Outport
  W2 : Outport  Port=2
  W3 : Outport  Port=3
  W4 : Outport  Port=4
  wires:
  W7/1(WPos) -> W4/1
  W6/1(WPos) -> W3/1
  W5/1(WPos) -> W2/1
  W/1(WPos) -> W1/1
  InW4/1 -> W7/1(WIn)
  InW3/1 -> W6/1(WIn)
  InW2/1 -> W5/1(WIn)
  InW1/1 -> W/1(WIn)

== system c00004M_harness/M141/S1 ==
  PhyMeasure : Inport
  SensorOut : Outport
  wires:
  PhyMeasure/1 -> SensorOut/1

== system c00004M_harness/M141/S2 ==
  PhyMeasure : Inport
  SensorOut : Outport
  wires:
  PhyMeasure/1 -> SensorOut/1

== system c00004M_harness/M141/S3 ==
  PhyMeasure : Inport
  SensorOut : Outport
  wires:
  PhyMeasure/1 -> SensorOut/1

== system c00004M_harness/M141/S4 ==
  PhyMeasure : Inport
  SensorOut : Outport
  wires:
  PhyMeasure/1 -> SensorOut/1

== system c00004M_harness/M142/Cyber ==
  note: Sensors
  note: Inputs For Window1
  note: Inputs for Window 2
  note: Inputs for window 3
  note: Inputs for window 4
  note: Users
  note: Users
  note: Sensors
  note: Users
  note: Sensors
  note: Users
  note: Sensors
  note: USERS
      | ---------------------------------
      | 0: None
      | 1: Ventana Arriba
      | 2: Ventana hasta arriba
      | 3: Ventana abajo
      | 4: Ventana hasta abajo
  note: 1: SUBE
      | 0: PARADO
      | -1 BAJA
  note: D = Driver (W1)
      | P1 = Passenger 1 (W2)
      | P2 = Passenger 2 (W3)
      | P3 = Passenger 3 (W4)
      | O = Obstacle
      | C = Control
      | Pri = Prioritizer
      | LD = LockDriver
      | PosW = PositionWindow
      | WL = WindowLogic
      | OW = ObstacleWindow
      | CWXC = ControlWindowXCentralized
      | S = Sensor
      | L = Lock
      | WPos = WindowPosition
      | M = Memory
      | InW = InputWindow
      | WIn = WindowInput
  PosW1 : Inport
  PosW2 : Inport  Port=2
  PosW3 : Inport  Port=3
  PosW4 : Inport  Port=4
  DW1 : Inport  Port=5
  DW3 : Inport  Port=6
  DW4 : Inport  Port=7
  P1W2 : Inport  Port=8
  P2W3 : Inport  Port=9
  P1W3 : Inport  Port=10
  P3W4 : Inport  Port=11
  P1W4 : Inport  Port=12
  OW1 : Inport  Port=13
  OW2 : Inport  Port=14
  OW3 : Inport  Port=15
  OW4 : Inport  Port=16
  CW1C : Inport  Port=17
  CW3C : Inport  Port=18
  CW4C : Inport  Port=19
  Pri1 : Subsystem
  Pri3 : Subsystem
  Pri4 : Subsystem
  WL : Subsystem
  WL1 : Subsystem
  WL2 : Subsystem
  WL3 : Subsystem
  W1 : Outport
  W2 : Outport  Port=2
  W3 : Outport  Port=3
  W4 : Outport  Port=4
  wires:
  CW4C/1 -> Pri4/4(CW4C)
  CW3C/1 -> Pri1/4(CW3C)
  CW1C/1 -> Pri3/2(CW1C)
  Pri3/1(User) -> WL/2(User)
  WL3/1(WindowLogicOutput) -> W4/1
  WL2/1(WindowLogicOutput) -> W3/1
  Pri4/1(User) -> WL3/2(User)
  OW4/1 -> WL3/3(OW)
  PosW4/1 -> WL3/1(WPos)
  P1W4/1 -> Pri4/3(P1)
  P3W4/1 -> Pri4/2(P)
  DW4/1 -> Pri4/1(D)
  P1W3/1 -> Pri1/3(P1)
  P2W3/1 -> Pri1/2(P)
  DW3/1 -> Pri1/1(D)
  OW3/1 -> WL2/3(OW)
  PosW3/1 -> WL2/1(WPos)
  Pri1/1(User) -> WL2/2(User)
  WL1/1(WindowLogicOutput) -> W2/1
  OW2/1 -> WL1/3(OW)
  PosW2/1 -> WL1/1(WPos)
  WL/1(WindowLogicOutput) -> W1/1
  DW1/1 -> Pri3/1(D)
  OW1/1 -> WL/3(OW)
  PosW1/1 -> WL/1(WPos)
  P1W2/1 -> WL1/2(User)

== system c00004M_harness/M142/Physical ==
  InW1 : Inport
  InW2 : Inport  Port=2
  InW3 : Inport  Port=3
  InW4 : Inport  Port=4
  W : Subsystem
  W5 : Subsystem
  W6 : Subsystem
  W7 : Subsystem
  W1 : Outport
  W2 : Outport  Port=2
  W3 : Outport  Port=3
  W4 : Outport  Port=4
  wires:
  W7/1(WPos) -> W4/1
  W6/1(WPos) -> W3/1
  W5/1(WPos) -> W2/1
  W/1(WPos) -> W1/1
  InW4/1 -> W7/1(WIn)
  InW3/1 -> W6/1(WIn)
  InW2/1 -> W5/1(WIn)
  InW1/1 -> W/1(WIn)

== system c00004M_harness/M142/S1 ==
  PhyMeasure : Inport
  SensorOut : Outport
  wires:
  PhyMeasure/1 -> SensorOut/1

== system c00004M_harness/M142/S2 ==
  PhyMeasure : Inport
  SensorOut : Outport
  wires:
  PhyMeasure/1 -> SensorOut/1

== system c00004M_harness/M142/S3 ==
  PhyMeasure : Inport
  SensorOut : Outport
  wires:
  PhyMeasure/1 -> SensorOut/1

== system c00004M_harness/M142/S4 ==
  PhyMeasure : Inport
  SensorOut : Outport
  wires:
  PhyMeasure/1 -> SensorOut/1

== system c00004M_harness/M143/Cyber ==
  note: Sensors
  note: Inputs For Window1
  note: Inputs for Window 2
  note: Inputs for window 3
  note: Inputs for window 4
  note: Users
  note: Users
  note: Sensors
  note: Users
  note: Sensors
  note: Users
  note: Sensors
  note: USERS
      | ---------------------------------
      | 0: None
      | 1: Ventana Arriba
      | 2: Ventana hasta arriba
      | 3: Ventana abajo
      | 4: Ventana hasta abajo
  note: 1: SUBE
      | 0: PARADO
      | -1 BAJA
  note: D = Driver (W1)
      | P1 = Passenger 1 (W2)
      | P2 = Passenger 2 (W3)
      | P3 = Passenger 3 (W4)
      | O = Obstacle
      | C = Control
      | Pri = Prioritizer
      | LD = LockDriver
      | PosW = PositionWindow
      | WL = WindowLogic
      | OW = ObstacleWindow
      | CWXC = ControlWindowXCentralized
      | S = Sensor
      | L = Lock
      | WPos = WindowPosition
      | M = Memory
      | InW = InputWindow
      | WIn = WindowInput
  PosW1 : Inport
  PosW2 : Inport  Port=2
  PosW3 : Inport  Port=3
  PosW4 : Inport  Port=4
  DW1 : Inport  Port=5
  DW3 : Inport  Port=6
  DW4 : Inport  Port=7
  P1W2 : Inport  Port=8
  P2W3 : Inport  Port=9
  P1W3 : Inport  Port=10
  P3W4 : Inport  Port=11
  P1W4 : Inport  Port=12
  OW1 : Inport  Port=13
  OW2 : Inport  Port=14
  OW3 : Inport  Port=15
  OW4 : Inport  Port=16
  CW1C : Inport  Port=17
  CW3C : Inport  Port=18
  CW4C : Inport  Port=19
  Pri1 : Subsystem
  Pri3 : Subsystem
  Pri4 : Subsystem
  WL : Subsystem
  WL1 : Subsystem
  WL2 : Subsystem
  WL3 : Subsystem
  W1 : Outport
  W2 : Outport  Port=2
  W3 : Outport  Port=3
  W4 : Outport  Port=4
  wires:
  CW4C/1 -> Pri4/4(CW4C)
  CW3C/1 -> Pri1/4(CW3C)
  CW1C/1 -> Pri3/2(CW1C)
  Pri3/1(User) -> WL/2(User)
  WL3/1(WindowLogicOutput) -> W4/1
  WL2/1(WindowLogicOutput) -> W3/1
  Pri4/1(User) -> WL3/2(User)
  OW4/1 -> WL3/3(OW)
  PosW4/1 -> WL3/1(WPos)
  P1W4/1 -> Pri4/3(P1)
  P3W4/1 -> Pri4/2(P)
  DW4/1 -> Pri4/1(D)
  P1W3/1 -> Pri1/3(P1)
  P2W3/1 -> Pri1/2(P)
  DW3/1 -> Pri1/1(D)
  OW3/1 -> WL2/3(OW)
  PosW3/1 -> WL2/1(WPos)
  Pri1/1(User) -> WL2/2(User)
  WL1/1(WindowLogicOutput) -> W2/1
  OW2/1 -> WL1/3(OW)
  PosW2/1 -> WL1/1(WPos)
  WL/1(WindowLogicOutput) -> W1/1
  DW1/1 -> Pri3/1(D)
  OW1/1 -> WL/3(OW)
  PosW1/1 -> WL/1(WPos)
  P1W2/1 -> WL1/2(User)

== system c00004M_harness/M143/Physical ==
  InW1 : Inport
  InW2 : Inport  Port=2
  InW3 : Inport  Port=3
  InW4 : Inport  Port=4
  W : Subsystem
  W5 : Subsystem
  W6 : Subsystem
  W7 : Subsystem
  W1 : Outport
  W2 : Outport  Port=2
  W3 : Outport  Port=3
  W4 : Outport  Port=4
  wires:
  W7/1(WPos) -> W4/1
  W6/1(WPos) -> W3/1
  W5/1(WPos) -> W2/1
  W/1(WPos) -> W1/1
  InW4/1 -> W7/1(WIn)
  InW3/1 -> W6/1(WIn)
  InW2/1 -> W5/1(WIn)
  InW1/1 -> W/1(WIn)

== system c00004M_harness/M143/S1 ==
  PhyMeasure : Inport
  SensorOut : Outport
  wires:
  PhyMeasure/1 -> SensorOut/1

== system c00004M_harness/M143/S2 ==
  PhyMeasure : Inport
  SensorOut : Outport
  wires:
  PhyMeasure/1 -> SensorOut/1

== system c00004M_harness/M143/S3 ==
  PhyMeasure : Inport
  SensorOut : Outport
  wires:
  PhyMeasure/1 -> SensorOut/1

== system c00004M_harness/M143/S4 ==
  PhyMeasure : Inport
  SensorOut : Outport
  wires:
  PhyMeasure/1 -> SensorOut/1

== system c00004M_harness/M144/Cyber ==
  note: Sensors
  note: Inputs For Window1
  note: Inputs for Window 2
  note: Inputs for window 3
  note: Inputs for window 4
  note: Users
  note: Users
  note: Sensors
  note: Users
  note: Sensors
  note: Users
  note: Sensors
  note: USERS
      | ---------------------------------
      | 0: None
      | 1: Ventana Arriba
      | 2: Ventana hasta arriba
      | 3: Ventana abajo
      | 4: Ventana hasta abajo
  note: 1: SUBE
      | 0: PARADO
      | -1 BAJA
  note: D = Driver (W1)
      | P1 = Passenger 1 (W2)
      | P2 = Passenger 2 (W3)
      | P3 = Passenger 3 (W4)
      | O = Obstacle
      | C = Control
      | Pri = Prioritizer
      | LD = LockDriver
      | PosW = PositionWindow
      | WL = WindowLogic
      | OW = ObstacleWindow
      | CWXC = ControlWindowXCentralized
      | S = Sensor
      | L = Lock
      | WPos = WindowPosition
      | M = Memory
      | InW = InputWindow
      | WIn = WindowInput
  PosW1 : Inport
  PosW2 : Inport  Port=2
  PosW3 : Inport  Port=3
  PosW4 : Inport  Port=4
  DW1 : Inport  Port=5
  DW3 : Inport  Port=6
  DW4 : Inport  Port=7
  P1W2 : Inport  Port=8
  P2W3 : Inport  Port=9
  P1W3 : Inport  Port=10
  P3W4 : Inport  Port=11
  P1W4 : Inport  Port=12
  OW1 : Inport  Port=13
  OW2 : Inport  Port=14
  OW3 : Inport  Port=15
  OW4 : Inport  Port=16
  CW1C : Inport  Port=17
  CW3C : Inport  Port=18
  CW4C : Inport  Port=19
  Pri1 : Subsystem
  Pri3 : Subsystem
  Pri4 : Subsystem
  WL : Subsystem
  WL1 : Subsystem
  WL2 : Subsystem
  WL3 : Subsystem
  W1 : Outport
  W2 : Outport  Port=2
  W3 : Outport  Port=3
  W4 : Outport  Port=4
  wires:
  CW4C/1 -> Pri4/4(CW4C)
  CW3C/1 -> Pri1/4(CW3C)
  CW1C/1 -> Pri3/2(CW1C)
  Pri3/1(User) -> WL/2(User)
  WL3/1(WindowLogicOutput) -> W4/1
  WL2/1(WindowLogicOutput) -> W3/1
  Pri4/1(User) -> WL3/2(User)
  OW4/1 -> WL3/3(OW)
  PosW4/1 -> WL3/1(WPos)
  P1W4/1 -> Pri4/3(P1)
  P3W4/1 -> Pri4/2(P)
  DW4/1 -> Pri4/1(D)
  P1W3/1 -> Pri1/3(P1)
  P2W3/1 -> Pri1/2(P)
  DW3/1 -> Pri1/1(D)
  OW3/1 -> WL2/3(OW)
  PosW3/1 -> WL2/1(WPos)
  Pri1/1(User) -> WL2/2(User)
  WL1/1(WindowLogicOutput) -> W2/1
  OW2/1 -> WL1/3(OW)
  PosW2/1 -> WL1/1(WPos)
  WL/1(WindowLogicOutput) -> W1/1
  DW1/1 -> Pri3/1(D)
  OW1/1 -> WL/3(OW)
  PosW1/1 -> WL/1(WPos)
  P1W2/1 -> WL1/2(User)

== system c00004M_harness/M144/Physical ==
  InW1 : Inport
  InW2 : Inport  Port=2
  InW3 : Inport  Port=3
  InW4 : Inport  Port=4
  W : Subsystem
  W5 : Subsystem
  W6 : Subsystem
  W7 : Subsystem
  W1 : Outport
  W2 : Outport  Port=2
  W3 : Outport  Port=3
  W4 : Outport  Port=4
  wires:
  W7/1(WPos) -> W4/1
  W6/1(WPos) -> W3/1
  W5/1(WPos) -> W2/1
  W/1(WPos) -> W1/1
  InW4/1 -> W7/1(WIn)
  InW3/1 -> W6/1(WIn)
  InW2/1 -> W5/1(WIn)
  InW1/1 -> W/1(WIn)

== system c00004M_harness/M144/S1 ==
  PhyMeasure : Inport
  SensorOut : Outport
  wires:
  PhyMeasure/1 -> SensorOut/1

== system c00004M_harness/M144/S2 ==
  PhyMeasure : Inport
  SensorOut : Outport
  wires:
  PhyMeasure/1 -> SensorOut/1

== system c00004M_harness/M144/S3 ==
  PhyMeasure : Inport
  SensorOut : Outport
  wires:
  PhyMeasure/1 -> SensorOut/1

== system c00004M_harness/M144/S4 ==
  PhyMeasure : Inport
  SensorOut : Outport
  wires:
  PhyMeasure/1 -> SensorOut/1

== system c00004M_harness/M145/Cyber ==
  note: Sensors
  note: Inputs For Window1
  note: Inputs for Window 2
  note: Inputs for window 3
  note: Inputs for window 4
  note: Users
  note: Users
  note: Sensors
  note: Users
  note: Sensors
  note: Users
  note: Sensors
  note: USERS
      | ---------------------------------
      | 0: None
      | 1: Ventana Arriba
      | 2: Ventana hasta arriba
      | 3: Ventana abajo
      | 4: Ventana hasta abajo
  note: 1: SUBE
      | 0: PARADO
      | -1 BAJA
  note: D = Driver (W1)
      | P1 = Passenger 1 (W2)
      | P2 = Passenger 2 (W3)
      | P3 = Passenger 3 (W4)
      | O = Obstacle
      | C = Control
      | Pri = Prioritizer
      | LD = LockDriver
      | PosW = PositionWindow
      | WL = WindowLogic
      | OW = ObstacleWindow
      | CWXC = ControlWindowXCentralized
      | S = Sensor
      | L = Lock
      | WPos = WindowPosition
      | M = Memory
      | InW = InputWindow
      | WIn = WindowInput
  PosW1 : Inport
  PosW2 : Inport  Port=2
  PosW3 : Inport  Port=3
  PosW4 : Inport  Port=4
  DW1 : Inport  Port=5
  DW3 : Inport  Port=6
  DW4 : Inport  Port=7
  P1W2 : Inport  Port=8
  P2W3 : Inport  Port=9
  P1W3 : Inport  Port=10
  P3W4 : Inport  Port=11
  P1W4 : Inport  Port=12
  OW1 : Inport  Port=13
  OW2 : Inport  Port=14
  OW3 : Inport  Port=15
  OW4 : Inport  Port=16
  CW1C : Inport  Port=17
  CW3C : Inport  Port=18
  CW4C : Inport  Port=19
  Pri1 : Subsystem
  Pri3 : Subsystem
  Pri4 : Subsystem
  WL : Subsystem
  WL1 : Subsystem
  WL2 : Subsystem
  WL3 : Subsystem
  W1 : Outport
  W2 : Outport  Port=2
  W3 : Outport  Port=3
  W4 : Outport  Port=4
  wires:
  CW4C/1 -> Pri4/4(CW4C)
  CW3C/1 -> Pri1/4(CW3C)
  CW1C/1 -> Pri3/2(CW1C)
  Pri3/1(User) -> WL/2(User)
  WL3/1(WindowLogicOutput) -> W4/1
  WL2/1(WindowLogicOutput) -> W3/1
  Pri4/1(User) -> WL3/2(User)
  OW4/1 -> WL3/3(OW)
  PosW4/1 -> WL3/1(WPos)
  P1W4/1 -> Pri4/3(P1)
  P3W4/1 -> Pri4/2(P)
  DW4/1 -> Pri4/1(D)
  P1W3/1 -> Pri1/3(P1)
  P2W3/1 -> Pri1/2(P)
  DW3/1 -> Pri1/1(D)
  OW3/1 -> WL2/3(OW)
  PosW3/1 -> WL2/1(WPos)
  Pri1/1(User) -> WL2/2(User)
  WL1/1(WindowLogicOutput) -> W2/1
  OW2/1 -> WL1/3(OW)
  PosW2/1 -> WL1/1(WPos)
  WL/1(WindowLogicOutput) -> W1/1
  DW1/1 -> Pri3/1(D)
  OW1/1 -> WL/3(OW)
  PosW1/1 -> WL/1(WPos)
  P1W2/1 -> WL1/2(User)

== system c00004M_harness/M145/Physical ==
  InW1 : Inport
  InW2 : Inport  Port=2
  InW3 : Inport  Port=3
  InW4 : Inport  Port=4
  W : Subsystem
  W5 : Subsystem
  W6 : Subsystem
  W7 : Subsystem
  W1 : Outport
  W2 : Outport  Port=2
  W3 : Outport  Port=3
  W4 : Outport  Port=4
  wires:
  W7/1(WPos) -> W4/1
  W6/1(WPos) -> W3/1
  W5/1(WPos) -> W2/1
  W/1(WPos) -> W1/1
  InW4/1 -> W7/1(WIn)
  InW3/1 -> W6/1(WIn)
  InW2/1 -> W5/1(WIn)
  InW1/1 -> W/1(WIn)

== system c00004M_harness/M145/S1 ==
  PhyMeasure : Inport
  SensorOut : Outport
  wires:
  PhyMeasure/1 -> SensorOut/1

== system c00004M_harness/M145/S2 ==
  PhyMeasure : Inport
  SensorOut : Outport
  wires:
  PhyMeasure/1 -> SensorOut/1

== system c00004M_harness/M145/S3 ==
  PhyMeasure : Inport
  SensorOut : Outport
  wires:
  PhyMeasure/1 -> SensorOut/1

== system c00004M_harness/M145/S4 ==
  PhyMeasure : Inport
  SensorOut : Outport
  wires:
  PhyMeasure/1 -> SensorOut/1

== system c00004M_harness/M146/Cyber ==
  note: Sensors
  note: Inputs For Window1
  note: Inputs for Window 2
  note: Inputs for window 3
  note: Inputs for window 4
  note: Users
  note: Users
  note: Sensors
  note: Users
  note: Sensors
  note: Users
  note: Sensors
  note: USERS
      | ---------------------------------
      | 0: None
      | 1: Ventana Arriba
      | 2: Ventana hasta arriba
      | 3: Ventana abajo
      | 4: Ventana hasta abajo
  note: 1: SUBE
      | 0: PARADO
      | -1 BAJA
  note: D = Driver (W1)
      | P1 = Passenger 1 (W2)
      | P2 = Passenger 2 (W3)
      | P3 = Passenger 3 (W4)
      | O = Obstacle
      | C = Control
      | Pri = Prioritizer
      | LD = LockDriver
      | PosW = PositionWindow
      | WL = WindowLogic
      | OW = ObstacleWindow
      | CWXC = ControlWindowXCentralized
      | S = Sensor
      | L = Lock
      | WPos = WindowPosition
      | M = Memory
      | InW = InputWindow
      | WIn = WindowInput
  PosW1 : Inport
  PosW2 : Inport  Port=2
  PosW3 : Inport  Port=3
  PosW4 : Inport  Port=4
  DW1 : Inport  Port=5
  DW3 : Inport  Port=6
  DW4 : Inport  Port=7
  P1W2 : Inport  Port=8
  P2W3 : Inport  Port=9
  P1W3 : Inport  Port=10
  P3W4 : Inport  Port=11
  P1W4 : Inport  Port=12
  OW1 : Inport  Port=13
  OW2 : Inport  Port=14
  OW3 : Inport  Port=15
  OW4 : Inport  Port=16
  CW1C : Inport  Port=17
  CW3C : Inport  Port=18
  CW4C : Inport  Port=19
  Pri1 : Subsystem
  Pri3 : Subsystem
  Pri4 : Subsystem
  WL : Subsystem
  WL1 : Subsystem
  WL2 : Subsystem
  WL3 : Subsystem
  W1 : Outport
  W2 : Outport  Port=2
  W3 : Outport  Port=3
  W4 : Outport  Port=4
  wires:
  CW4C/1 -> Pri4/4(CW4C)
  CW3C/1 -> Pri1/4(CW3C)
  CW1C/1 -> Pri3/2(CW1C)
  Pri3/1(User) -> WL/2(User)
  WL3/1(WindowLogicOutput) -> W4/1
  WL2/1(WindowLogicOutput) -> W3/1
  Pri4/1(User) -> WL3/2(User)
  OW4/1 -> WL3/3(OW)
  PosW4/1 -> WL3/1(WPos)
  P1W4/1 -> Pri4/3(P1)
  P3W4/1 -> Pri4/2(P)
  DW4/1 -> Pri4/1(D)
  P1W3/1 -> Pri1/3(P1)
  P2W3/1 -> Pri1/2(P)
  DW3/1 -> Pri1/1(D)
  OW3/1 -> WL2/3(OW)
  PosW3/1 -> WL2/1(WPos)
  Pri1/1(User) -> WL2/2(User)
  WL1/1(WindowLogicOutput) -> W2/1
  OW2/1 -> WL1/3(OW)
  PosW2/1 -> WL1/1(WPos)
  WL/1(WindowLogicOutput) -> W1/1
  DW1/1 -> Pri3/1(D)
  OW1/1 -> WL/3(OW)
  PosW1/1 -> WL/1(WPos)
  P1W2/1 -> WL1/2(User)

== system c00004M_harness/M146/Physical ==
  InW1 : Inport
  InW2 : Inport  Port=2
  InW3 : Inport  Port=3
  InW4 : Inport  Port=4
  W : Subsystem
  W5 : Subsystem
  W6 : Subsystem
  W7 : Subsystem
  W1 : Outport
  W2 : Outport  Port=2
  W3 : Outport  Port=3
  W4 : Outport  Port=4
  wires:
  W7/1(WPos) -> W4/1
  W6/1(WPos) -> W3/1
  W5/1(WPos) -> W2/1
  W/1(WPos) -> W1/1
  InW4/1 -> W7/1(WIn)
  InW3/1 -> W6/1(WIn)
  InW2/1 -> W5/1(WIn)
  InW1/1 -> W/1(WIn)

== system c00004M_harness/M146/S1 ==
  PhyMeasure : Inport
  SensorOut : Outport
  wires:
  PhyMeasure/1 -> SensorOut/1

== system c00004M_harness/M146/S2 ==
  PhyMeasure : Inport
  SensorOut : Outport
  wires:
  PhyMeasure/1 -> SensorOut/1

== system c00004M_harness/M146/S3 ==
  PhyMeasure : Inport
  SensorOut : Outport
  wires:
  PhyMeasure/1 -> SensorOut/1

== system c00004M_harness/M146/S4 ==
  PhyMeasure : Inport
  SensorOut : Outport
  wires:
  PhyMeasure/1 -> SensorOut/1

== system c00004M_harness/M147/Cyber ==
  note: Sensors
  note: Inputs For Window1
  note: Inputs for Window 2
  note: Inputs for window 3
  note: Inputs for window 4
  note: Users
  note: Users
  note: Sensors
  note: Users
  note: Sensors
  note: Users
  note: Sensors
  note: USERS
      | ---------------------------------
      | 0: None
      | 1: Ventana Arriba
      | 2: Ventana hasta arriba
      | 3: Ventana abajo
      | 4: Ventana hasta abajo
  note: 1: SUBE
      | 0: PARADO
      | -1 BAJA
  note: D = Driver (W1)
      | P1 = Passenger 1 (W2)
      | P2 = Passenger 2 (W3)
      | P3 = Passenger 3 (W4)
      | O = Obstacle
      | C = Control
      | Pri = Prioritizer
      | LD = LockDriver
      | PosW = PositionWindow
      | WL = WindowLogic
      | OW = ObstacleWindow
      | CWXC = ControlWindowXCentralized
      | S = Sensor
      | L = Lock
      | WPos = WindowPosition
      | M = Memory
      | InW = InputWindow
      | WIn = WindowInput
  PosW1 : Inport
  PosW2 : Inport  Port=2
  PosW3 : Inport  Port=3
  PosW4 : Inport  Port=4
  DW1 : Inport  Port=5
  DW3 : Inport  Port=6
  DW4 : Inport  Port=7
  P1W2 : Inport  Port=8
  P2W3 : Inport  Port=9
  P1W3 : Inport  Port=10
  P3W4 : Inport  Port=11
  P1W4 : Inport  Port=12
  OW1 : Inport  Port=13
  OW2 : Inport  Port=14
  OW3 : Inport  Port=15
  OW4 : Inport  Port=16
  CW1C : Inport  Port=17
  CW3C : Inport  Port=18
  CW4C : Inport  Port=19
  Pri1 : Subsystem
  Pri3 : Subsystem
  Pri4 : Subsystem
  WL : Subsystem
  WL1 : Subsystem
  WL2 : Subsystem
  WL3 : Subsystem
  W1 : Outport
  W2 : Outport  Port=2
  W3 : Outport  Port=3
  W4 : Outport  Port=4
  wires:
  CW4C/1 -> Pri4/4(CW4C)
  CW3C/1 -> Pri1/4(CW3C)
  CW1C/1 -> Pri3/2(CW1C)
  Pri3/1(User) -> WL/2(User)
  WL3/1(WindowLogicOutput) -> W4/1
  WL2/1(WindowLogicOutput) -> W3/1
  Pri4/1(User) -> WL3/2(User)
  OW4/1 -> WL3/3(OW)
  PosW4/1 -> WL3/1(WPos)
  P1W4/1 -> Pri4/3(P1)
  P3W4/1 -> Pri4/2(P)
  DW4/1 -> Pri4/1(D)
  P1W3/1 -> Pri1/3(P1)
  P2W3/1 -> Pri1/2(P)
  DW3/1 -> Pri1/1(D)
  OW3/1 -> WL2/3(OW)
  PosW3/1 -> WL2/1(WPos)
  Pri1/1(User) -> WL2/2(User)
  WL1/1(WindowLogicOutput) -> W2/1
  OW2/1 -> WL1/3(OW)
  PosW2/1 -> WL1/1(WPos)
  WL/1(WindowLogicOutput) -> W1/1
  DW1/1 -> Pri3/1(D)
  OW1/1 -> WL/3(OW)
  PosW1/1 -> WL/1(WPos)
  P1W2/1 -> WL1/2(User)

== system c00004M_harness/M147/Physical ==
  InW1 : Inport
  InW2 : Inport  Port=2
  InW3 : Inport  Port=3
  InW4 : Inport  Port=4
  W : Subsystem
  W5 : Subsystem
  W6 : Subsystem
  W7 : Subsystem
  W1 : Outport
  W2 : Outport  Port=2
  W3 : Outport  Port=3
  W4 : Outport  Port=4
  wires:
  W7/1(WPos) -> W4/1
  W6/1(WPos) -> W3/1
  W5/1(WPos) -> W2/1
  W/1(WPos) -> W1/1
  InW4/1 -> W7/1(WIn)
  InW3/1 -> W6/1(WIn)
  InW2/1 -> W5/1(WIn)
  InW1/1 -> W/1(WIn)

== system c00004M_harness/M147/S1 ==
  PhyMeasure : Inport
  SensorOut : Outport
  wires:
  PhyMeasure/1 -> SensorOut/1

== system c00004M_harness/M147/S2 ==
  PhyMeasure : Inport
  SensorOut : Outport
  wires:
  PhyMeasure/1 -> SensorOut/1

== system c00004M_harness/M147/S3 ==
  PhyMeasure : Inport
  SensorOut : Outport
  wires:
  PhyMeasure/1 -> SensorOut/1

== system c00004M_harness/M147/S4 ==
  PhyMeasure : Inport
  SensorOut : Outport
  wires:
  PhyMeasure/1 -> SensorOut/1
